simulink model "P_controller_DIFFERENT_KP_2ORDER"  (R2023b)
settings: Solver=VariableStepAuto  StartTime=0.0  StopTime=10.0  RelTol=1e-3
settings Model: Creator=ascom  LastModifiedBy=ascom

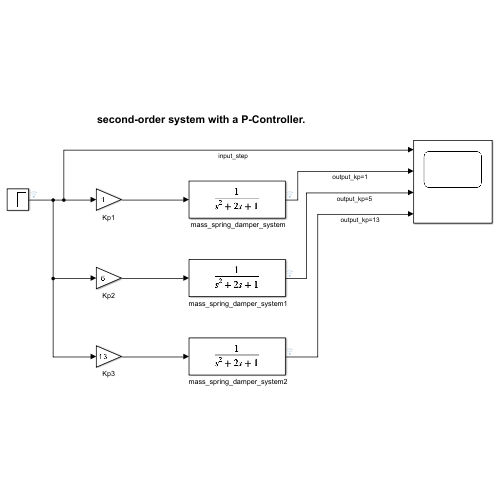
[thumbnail: Simulink's stored preview of the top-level diagram]
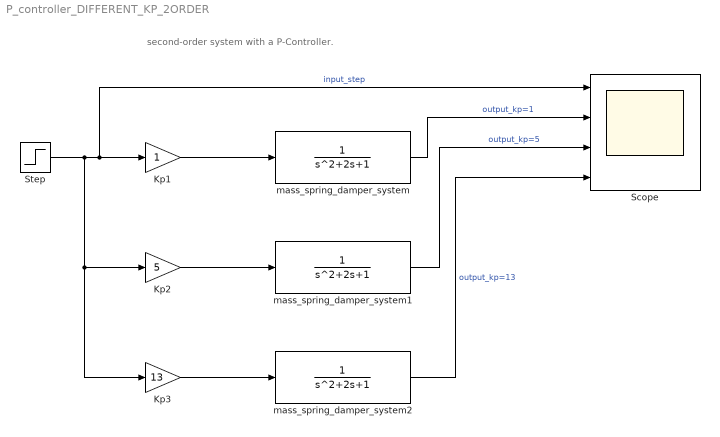
== system P_controller_DIFFERENT_KP_2ORDER ==
  note: second-order system with a P-Controller.
  " mass_spring_damper_system" : TransferFcn
  " mass_spring_damper_system1" : TransferFcn
  " mass_spring_damper_system2" : TransferFcn
  Kp1 : Gain
  Kp2 : Gain  Gain=5
  Kp3 : Gain  Gain=13
  Scope : Scope  NumInputPorts=4
  Step : Step  SampleTime=0
  wires:
  Kp1/1 -> " mass_spring_damper_system"/1
  " mass_spring_damper_system"/1 -> Scope/2  "output_kp=1"
  " mass_spring_damper_system1"/1 -> Scope/3  "output_kp=5"
  Kp2/1 -> " mass_spring_damper_system1"/1
  Kp3/1 -> " mass_spring_damper_system2"/1
  Step/1 -> Kp3/1, Kp2/1, Scope/1, Kp1/1  "input_step"
  " mass_spring_damper_system2"/1 -> Scope/4  "output_kp=13"
